simulink model "Ej_2_2"  (R2022b)
settings: Solver=VariableStepAuto  StartTime=0.0  StopTime=4000  RelTol=1e-3
settings Model: Creator=rrilo  LastModifiedBy=rrilo

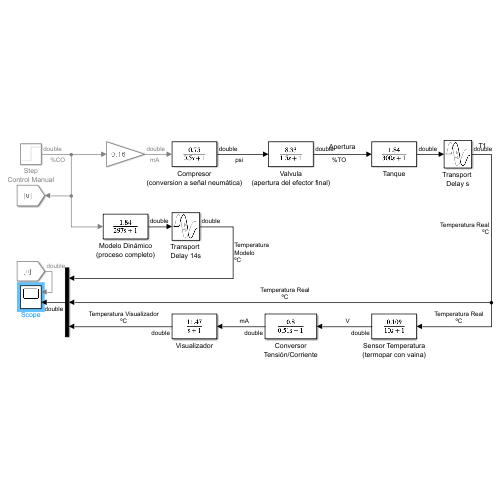
[thumbnail: Simulink's stored preview of the top-level diagram]
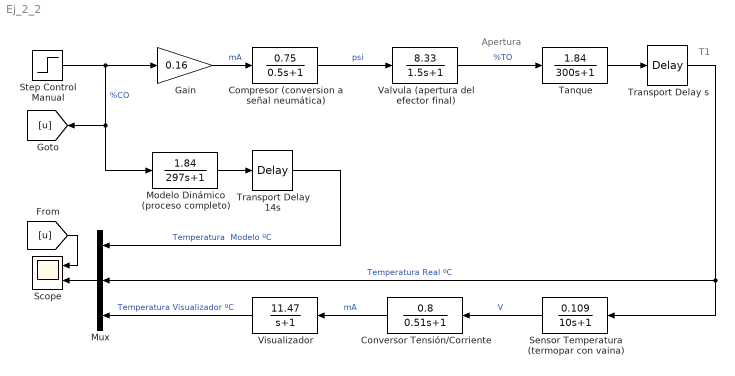
== system Ej_2_2 ==
  note: T1
  note: Apertura
  Compresor (conversion a señal neumática) : TransferFcn  Numerator=[0.75]  Denominator=[0.5 1]
  Conversor Tensión/Corriente : TransferFcn  Numerator=[0.8]  Denominator=[0.51 1]
  Gain : Gain  Gain=0.16
  Modelo Dinámico (proceso completo) : TransferFcn  Numerator=[1.84]  Denominator=[297 1]
  Mux : Mux  Inputs=3
  Scope : Scope  NumInputPorts=2
  Sensor Temperatura (termopar con vaina) : TransferFcn  Numerator=[0.109]  Denominator=[10 1]
  Step Control Manual : Step  After=54.34  SampleTime=0
  Tanque : TransferFcn  Numerator=[1.84]  Denominator=[300 1]
  Transport Delay 14s : TransportDelay  DelayTime=14
  Transport Delay s : TransportDelay
  Valvula (apertura del efector final) : TransferFcn  Numerator=[8.33]  Denominator=[1.5 1]
  Visualizador : TransferFcn  Numerator=[11.47]  Denominator=[1 1]
  wires:
  Tanque/1 -> Transport Delay s/1
  Modelo Dinámico (proceso completo)/1 -> Transport Delay 14s/1
  Gain/1 -> Compresor (conversion a señal neumática)/1  "mA"
  Step Control Manual/1 -> [u], Modelo Dinámico (proceso completo)/1, Gain/1  "%CO"
  Compresor (conversion a señal neumática)/1 -> Valvula (apertura del efector final)/1  "psi"
  Valvula (apertura del efector final)/1 -> Tanque/1  "%TO"
  Mux/1 -> Scope/2
  Conversor Tensión/Corriente/1 -> Visualizador/1  "mA"
  Sensor Temperatura (termopar con vaina)/1 -> Conversor Tensión/Corriente/1  "V"
  Transport Delay s/1 -> Sensor Temperatura (termopar con vaina)/1, Mux/2  "Temperatura Real ºC"
  Transport Delay 14s/1 -> Mux/1  "Temperatura  Modelo ºC"
  Visualizador/1 -> Mux/3  "Temperatura Visualizador ºC"
  [u] -> Scope/1
